simulink model "pattern3x3_training_2023clock"  (R2024a)
settings: Solver=FixedStepAuto  StartTime=0.0  StopTime=2  FixedStep=0.000005  RelTol=1e-3
model workspace (MAT data in the model file):
  part1_v1 = 1
values from neighbouring files (symbols this model uses):
  full_pattern = load('Pattern4_250.CSV')    [model_setup4.m]
  max_weight2 = 255    [model_setup4.m]
  min_weight2 = 150    [model_setup4.m]
  Th_minus_count2 = 10    [model_setup4.m]    (also in model_setup_test.m = 5)
  Th_plus_count2 = 20    [model_setup4.m]    (also in model_setup_test.m)
libraries: simulink x1
(part 7 of 9)

== system pattern3x3_training_2023clock/Synapse33/Clock3 ==
  clock : Inport
  "Reset " : Inport  Port=2
  Memory2 : Memory
  NOT1 : Logic  Operator=NOT  IconShape=distinctive  AllPortsSameDT=off  OutDataTypeStr=boolean
  Product1 : Product
  Triggered Subsystem1 : Subsystem  TreatAsAtomicUnit=on
  T : Outport  VectorParamsAs1DForOutWhenUnconnected=off
  wires:
  Memory2/1 -> Triggered Subsystem1/1(In1)
  Product1/1 -> T/1, Memory2/1
  "Reset "/1 -> NOT1/1
  Triggered Subsystem1/1(Out1) -> Product1/1
  NOT1/1 -> Product1/2
  clock/1 -> Triggered Subsystem1/Trigger

== system pattern3x3_training_2023clock/Synapse33/Subsystem ==
  delta_weight : Inport
  before_weight : Inport  Port=2
  Trigger : TriggerPort  VariantControl=(inherit)  PortDimensions=1
  Sum : Sum  Inputs=|++
  weight : Outport
  wires:
  delta_weight/1 -> Sum/1
  Sum/1 -> weight/1
  before_weight/1 -> Sum/2

== system pattern3x3_training_2023clock/Synapse34/Clock1 ==
  clock : Inport
  "Reset " : Inport  Port=2
  Memory2 : Memory
  NOT1 : Logic  Operator=NOT  IconShape=distinctive  AllPortsSameDT=off  OutDataTypeStr=boolean
  Product1 : Product
  Triggered Subsystem1 : Subsystem  TreatAsAtomicUnit=on
  T : Outport  VectorParamsAs1DForOutWhenUnconnected=off
  wires:
  Memory2/1 -> Triggered Subsystem1/1(In1)
  Product1/1 -> T/1, Memory2/1
  "Reset "/1 -> NOT1/1
  Triggered Subsystem1/1(Out1) -> Product1/1
  NOT1/1 -> Product1/2
  clock/1 -> Triggered Subsystem1/Trigger

== system pattern3x3_training_2023clock/Synapse34/Clock2 ==
  clock : Inport
  "Reset " : Inport  Port=2
  Memory2 : Memory
  NOT1 : Logic  Operator=NOT  IconShape=distinctive  AllPortsSameDT=off  OutDataTypeStr=boolean
  Product1 : Product
  Triggered Subsystem1 : Subsystem  TreatAsAtomicUnit=on
  T : Outport  VectorParamsAs1DForOutWhenUnconnected=off
  wires:
  Memory2/1 -> Triggered Subsystem1/1(In1)
  Product1/1 -> T/1, Memory2/1
  "Reset "/1 -> NOT1/1
  Triggered Subsystem1/1(Out1) -> Product1/1
  NOT1/1 -> Product1/2
  clock/1 -> Triggered Subsystem1/Trigger

== system pattern3x3_training_2023clock/Synapse34/Clock3 ==
  clock : Inport
  "Reset " : Inport  Port=2
  Memory2 : Memory
  NOT1 : Logic  Operator=NOT  IconShape=distinctive  AllPortsSameDT=off  OutDataTypeStr=boolean
  Product1 : Product
  Triggered Subsystem1 : Subsystem  TreatAsAtomicUnit=on
  T : Outport  VectorParamsAs1DForOutWhenUnconnected=off
  wires:
  Memory2/1 -> Triggered Subsystem1/1(In1)
  Product1/1 -> T/1, Memory2/1
  "Reset "/1 -> NOT1/1
  Triggered Subsystem1/1(Out1) -> Product1/1
  NOT1/1 -> Product1/2
  clock/1 -> Triggered Subsystem1/Trigger

== system pattern3x3_training_2023clock/Synapse34/Subsystem ==
  delta_weight : Inport
  before_weight : Inport  Port=2
  Trigger : TriggerPort  VariantControl=(inherit)  PortDimensions=1
  Sum : Sum  Inputs=|++
  weight : Outport
  wires:
  delta_weight/1 -> Sum/1
  Sum/1 -> weight/1
  before_weight/1 -> Sum/2

== system pattern3x3_training_2023clock/Synapse35/Clock1 ==
  clock : Inport
  "Reset " : Inport  Port=2
  Memory2 : Memory
  NOT1 : Logic  Operator=NOT  IconShape=distinctive  AllPortsSameDT=off  OutDataTypeStr=boolean
  Product1 : Product
  Triggered Subsystem1 : Subsystem  TreatAsAtomicUnit=on
  T : Outport  VectorParamsAs1DForOutWhenUnconnected=off
  wires:
  Memory2/1 -> Triggered Subsystem1/1(In1)
  Product1/1 -> T/1, Memory2/1
  "Reset "/1 -> NOT1/1
  Triggered Subsystem1/1(Out1) -> Product1/1
  NOT1/1 -> Product1/2
  clock/1 -> Triggered Subsystem1/Trigger

== system pattern3x3_training_2023clock/Synapse35/Clock2 ==
  clock : Inport
  "Reset " : Inport  Port=2
  Memory2 : Memory
  NOT1 : Logic  Operator=NOT  IconShape=distinctive  AllPortsSameDT=off  OutDataTypeStr=boolean
  Product1 : Product
  Triggered Subsystem1 : Subsystem  TreatAsAtomicUnit=on
  T : Outport  VectorParamsAs1DForOutWhenUnconnected=off
  wires:
  Memory2/1 -> Triggered Subsystem1/1(In1)
  Product1/1 -> T/1, Memory2/1
  "Reset "/1 -> NOT1/1
  Triggered Subsystem1/1(Out1) -> Product1/1
  NOT1/1 -> Product1/2
  clock/1 -> Triggered Subsystem1/Trigger

== system pattern3x3_training_2023clock/Synapse35/Clock3 ==
  clock : Inport
  "Reset " : Inport  Port=2
  Memory2 : Memory
  NOT1 : Logic  Operator=NOT  IconShape=distinctive  AllPortsSameDT=off  OutDataTypeStr=boolean
  Product1 : Product
  Triggered Subsystem1 : Subsystem  TreatAsAtomicUnit=on
  T : Outport  VectorParamsAs1DForOutWhenUnconnected=off
  wires:
  Memory2/1 -> Triggered Subsystem1/1(In1)
  Product1/1 -> T/1, Memory2/1
  "Reset "/1 -> NOT1/1
  Triggered Subsystem1/1(Out1) -> Product1/1
  NOT1/1 -> Product1/2
  clock/1 -> Triggered Subsystem1/Trigger

== system pattern3x3_training_2023clock/Synapse35/Subsystem ==
  delta_weight : Inport
  before_weight : Inport  Port=2
  Trigger : TriggerPort  VariantControl=(inherit)  PortDimensions=1
  Sum : Sum  Inputs=|++
  weight : Outport
  wires:
  delta_weight/1 -> Sum/1
  Sum/1 -> weight/1
  before_weight/1 -> Sum/2

== system pattern3x3_training_2023clock/Synapse36/Clock1 ==
  clock : Inport
  "Reset " : Inport  Port=2
  Memory2 : Memory
  NOT1 : Logic  Operator=NOT  IconShape=distinctive  AllPortsSameDT=off  OutDataTypeStr=boolean
  Product1 : Product
  Triggered Subsystem1 : Subsystem  TreatAsAtomicUnit=on
  T : Outport  VectorParamsAs1DForOutWhenUnconnected=off
  wires:
  Memory2/1 -> Triggered Subsystem1/1(In1)
  Product1/1 -> T/1, Memory2/1
  "Reset "/1 -> NOT1/1
  Triggered Subsystem1/1(Out1) -> Product1/1
  NOT1/1 -> Product1/2
  clock/1 -> Triggered Subsystem1/Trigger

== system pattern3x3_training_2023clock/Synapse36/Clock2 ==
  clock : Inport
  "Reset " : Inport  Port=2
  Memory2 : Memory
  NOT1 : Logic  Operator=NOT  IconShape=distinctive  AllPortsSameDT=off  OutDataTypeStr=boolean
  Product1 : Product
  Triggered Subsystem1 : Subsystem  TreatAsAtomicUnit=on
  T : Outport  VectorParamsAs1DForOutWhenUnconnected=off
  wires:
  Memory2/1 -> Triggered Subsystem1/1(In1)
  Product1/1 -> T/1, Memory2/1
  "Reset "/1 -> NOT1/1
  Triggered Subsystem1/1(Out1) -> Product1/1
  NOT1/1 -> Product1/2
  clock/1 -> Triggered Subsystem1/Trigger

== system pattern3x3_training_2023clock/Synapse36/Clock3 ==
  clock : Inport
  "Reset " : Inport  Port=2
  Memory2 : Memory
  NOT1 : Logic  Operator=NOT  IconShape=distinctive  AllPortsSameDT=off  OutDataTypeStr=boolean
  Product1 : Product
  Triggered Subsystem1 : Subsystem  TreatAsAtomicUnit=on
  T : Outport  VectorParamsAs1DForOutWhenUnconnected=off
  wires:
  Memory2/1 -> Triggered Subsystem1/1(In1)
  Product1/1 -> T/1, Memory2/1
  "Reset "/1 -> NOT1/1
  Triggered Subsystem1/1(Out1) -> Product1/1
  NOT1/1 -> Product1/2
  clock/1 -> Triggered Subsystem1/Trigger

== system pattern3x3_training_2023clock/Synapse36/Subsystem ==
  delta_weight : Inport
  before_weight : Inport  Port=2
  Trigger : TriggerPort  VariantControl=(inherit)  PortDimensions=1
  Sum : Sum  Inputs=|++
  weight : Outport
  wires:
  delta_weight/1 -> Sum/1
  Sum/1 -> weight/1
  before_weight/1 -> Sum/2

== system pattern3x3_training_2023clock/Synapse4/Clock1 ==
  clock : Inport
  "Reset " : Inport  Port=2
  Memory2 : Memory
  NOT1 : Logic  Operator=NOT  IconShape=distinctive  AllPortsSameDT=off  OutDataTypeStr=boolean
  Product1 : Product
  Triggered Subsystem1 : Subsystem  TreatAsAtomicUnit=on
  T : Outport  VectorParamsAs1DForOutWhenUnconnected=off
  wires:
  Memory2/1 -> Triggered Subsystem1/1(In1)
  Product1/1 -> T/1, Memory2/1
  "Reset "/1 -> NOT1/1
  Triggered Subsystem1/1(Out1) -> Product1/1
  NOT1/1 -> Product1/2
  clock/1 -> Triggered Subsystem1/Trigger

== system pattern3x3_training_2023clock/Synapse4/Clock2 ==
  clock : Inport
  "Reset " : Inport  Port=2
  Memory2 : Memory
  NOT1 : Logic  Operator=NOT  IconShape=distinctive  AllPortsSameDT=off  OutDataTypeStr=boolean
  Product1 : Product
  Triggered Subsystem1 : Subsystem  TreatAsAtomicUnit=on
  T : Outport  VectorParamsAs1DForOutWhenUnconnected=off
  wires:
  Memory2/1 -> Triggered Subsystem1/1(In1)
  Product1/1 -> T/1, Memory2/1
  "Reset "/1 -> NOT1/1
  Triggered Subsystem1/1(Out1) -> Product1/1
  NOT1/1 -> Product1/2
  clock/1 -> Triggered Subsystem1/Trigger

== system pattern3x3_training_2023clock/Synapse4/Clock3 ==
  clock : Inport
  "Reset " : Inport  Port=2
  Memory2 : Memory
  NOT1 : Logic  Operator=NOT  IconShape=distinctive  AllPortsSameDT=off  OutDataTypeStr=boolean
  Product1 : Product
  Triggered Subsystem1 : Subsystem  TreatAsAtomicUnit=on
  T : Outport  VectorParamsAs1DForOutWhenUnconnected=off
  wires:
  Memory2/1 -> Triggered Subsystem1/1(In1)
  Product1/1 -> T/1, Memory2/1
  "Reset "/1 -> NOT1/1
  Triggered Subsystem1/1(Out1) -> Product1/1
  NOT1/1 -> Product1/2
  clock/1 -> Triggered Subsystem1/Trigger

== system pattern3x3_training_2023clock/Synapse4/Subsystem ==
  delta_weight : Inport
  before_weight : Inport  Port=2
  Trigger : TriggerPort  VariantControl=(inherit)  PortDimensions=1
  Sum : Sum  Inputs=|++
  weight : Outport
  wires:
  delta_weight/1 -> Sum/1
  Sum/1 -> weight/1
  before_weight/1 -> Sum/2

== system pattern3x3_training_2023clock/Synapse5/Clock1 ==
  clock : Inport
  "Reset " : Inport  Port=2
  Memory2 : Memory
  NOT1 : Logic  Operator=NOT  IconShape=distinctive  AllPortsSameDT=off  OutDataTypeStr=boolean
  Product1 : Product
  Triggered Subsystem1 : Subsystem  TreatAsAtomicUnit=on
  T : Outport  VectorParamsAs1DForOutWhenUnconnected=off
  wires:
  Memory2/1 -> Triggered Subsystem1/1(In1)
  Product1/1 -> T/1, Memory2/1
  "Reset "/1 -> NOT1/1
  Triggered Subsystem1/1(Out1) -> Product1/1
  NOT1/1 -> Product1/2
  clock/1 -> Triggered Subsystem1/Trigger

== system pattern3x3_training_2023clock/Synapse5/Clock2 ==
  clock : Inport
  "Reset " : Inport  Port=2
  Memory2 : Memory
  NOT1 : Logic  Operator=NOT  IconShape=distinctive  AllPortsSameDT=off  OutDataTypeStr=boolean
  Product1 : Product
  Triggered Subsystem1 : Subsystem  TreatAsAtomicUnit=on
  T : Outport  VectorParamsAs1DForOutWhenUnconnected=off
  wires:
  Memory2/1 -> Triggered Subsystem1/1(In1)
  Product1/1 -> T/1, Memory2/1
  "Reset "/1 -> NOT1/1
  Triggered Subsystem1/1(Out1) -> Product1/1
  NOT1/1 -> Product1/2
  clock/1 -> Triggered Subsystem1/Trigger

== system pattern3x3_training_2023clock/Synapse5/Clock3 ==
  clock : Inport
  "Reset " : Inport  Port=2
  Memory2 : Memory
  NOT1 : Logic  Operator=NOT  IconShape=distinctive  AllPortsSameDT=off  OutDataTypeStr=boolean
  Product1 : Product
  Triggered Subsystem1 : Subsystem  TreatAsAtomicUnit=on
  T : Outport  VectorParamsAs1DForOutWhenUnconnected=off
  wires:
  Memory2/1 -> Triggered Subsystem1/1(In1)
  Product1/1 -> T/1, Memory2/1
  "Reset "/1 -> NOT1/1
  Triggered Subsystem1/1(Out1) -> Product1/1
  NOT1/1 -> Product1/2
  clock/1 -> Triggered Subsystem1/Trigger

== system pattern3x3_training_2023clock/Synapse5/Subsystem ==
  delta_weight : Inport
  before_weight : Inport  Port=2
  Trigger : TriggerPort  VariantControl=(inherit)  PortDimensions=1
  Sum : Sum  Inputs=|++
  weight : Outport
  wires:
  delta_weight/1 -> Sum/1
  Sum/1 -> weight/1
  before_weight/1 -> Sum/2

== system pattern3x3_training_2023clock/Synapse6/Clock1 ==
  clock : Inport
  "Reset " : Inport  Port=2
  Memory2 : Memory
  NOT1 : Logic  Operator=NOT  IconShape=distinctive  AllPortsSameDT=off  OutDataTypeStr=boolean
  Product1 : Product
  Triggered Subsystem1 : Subsystem  TreatAsAtomicUnit=on
  T : Outport  VectorParamsAs1DForOutWhenUnconnected=off
  wires:
  Memory2/1 -> Triggered Subsystem1/1(In1)
  Product1/1 -> T/1, Memory2/1
  "Reset "/1 -> NOT1/1
  Triggered Subsystem1/1(Out1) -> Product1/1
  NOT1/1 -> Product1/2
  clock/1 -> Triggered Subsystem1/Trigger

== system pattern3x3_training_2023clock/Synapse6/Clock2 ==
  clock : Inport
  "Reset " : Inport  Port=2
  Memory2 : Memory
  NOT1 : Logic  Operator=NOT  IconShape=distinctive  AllPortsSameDT=off  OutDataTypeStr=boolean
  Product1 : Product
  Triggered Subsystem1 : Subsystem  TreatAsAtomicUnit=on
  T : Outport  VectorParamsAs1DForOutWhenUnconnected=off
  wires:
  Memory2/1 -> Triggered Subsystem1/1(In1)
  Product1/1 -> T/1, Memory2/1
  "Reset "/1 -> NOT1/1
  Triggered Subsystem1/1(Out1) -> Product1/1
  NOT1/1 -> Product1/2
  clock/1 -> Triggered Subsystem1/Trigger

== system pattern3x3_training_2023clock/Synapse6/Clock3 ==
  clock : Inport
  "Reset " : Inport  Port=2
  Memory2 : Memory
  NOT1 : Logic  Operator=NOT  IconShape=distinctive  AllPortsSameDT=off  OutDataTypeStr=boolean
  Product1 : Product
  Triggered Subsystem1 : Subsystem  TreatAsAtomicUnit=on
  T : Outport  VectorParamsAs1DForOutWhenUnconnected=off
  wires:
  Memory2/1 -> Triggered Subsystem1/1(In1)
  Product1/1 -> T/1, Memory2/1
  "Reset "/1 -> NOT1/1
  Triggered Subsystem1/1(Out1) -> Product1/1
  NOT1/1 -> Product1/2
  clock/1 -> Triggered Subsystem1/Trigger

== system pattern3x3_training_2023clock/Synapse6/Subsystem ==
  delta_weight : Inport
  before_weight : Inport  Port=2
  Trigger : TriggerPort  VariantControl=(inherit)  PortDimensions=1
  Sum : Sum  Inputs=|++
  weight : Outport
  wires:
  delta_weight/1 -> Sum/1
  Sum/1 -> weight/1
  before_weight/1 -> Sum/2

== system pattern3x3_training_2023clock/Synapse7/Clock1 ==
  clock : Inport
  "Reset " : Inport  Port=2
  Memory2 : Memory
  NOT1 : Logic  Operator=NOT  IconShape=distinctive  AllPortsSameDT=off  OutDataTypeStr=boolean
  Product1 : Product
  Triggered Subsystem1 : Subsystem  TreatAsAtomicUnit=on
  T : Outport  VectorParamsAs1DForOutWhenUnconnected=off
  wires:
  Memory2/1 -> Triggered Subsystem1/1(In1)
  Product1/1 -> T/1, Memory2/1
  "Reset "/1 -> NOT1/1
  Triggered Subsystem1/1(Out1) -> Product1/1
  NOT1/1 -> Product1/2
  clock/1 -> Triggered Subsystem1/Trigger

== system pattern3x3_training_2023clock/Synapse7/Clock2 ==
  clock : Inport
  "Reset " : Inport  Port=2
  Memory2 : Memory
  NOT1 : Logic  Operator=NOT  IconShape=distinctive  AllPortsSameDT=off  OutDataTypeStr=boolean
  Product1 : Product
  Triggered Subsystem1 : Subsystem  TreatAsAtomicUnit=on
  T : Outport  VectorParamsAs1DForOutWhenUnconnected=off
  wires:
  Memory2/1 -> Triggered Subsystem1/1(In1)
  Product1/1 -> T/1, Memory2/1
  "Reset "/1 -> NOT1/1
  Triggered Subsystem1/1(Out1) -> Product1/1
  NOT1/1 -> Product1/2
  clock/1 -> Triggered Subsystem1/Trigger

== system pattern3x3_training_2023clock/Synapse7/Clock3 ==
  clock : Inport
  "Reset " : Inport  Port=2
  Memory2 : Memory
  NOT1 : Logic  Operator=NOT  IconShape=distinctive  AllPortsSameDT=off  OutDataTypeStr=boolean
  Product1 : Product
  Triggered Subsystem1 : Subsystem  TreatAsAtomicUnit=on
  T : Outport  VectorParamsAs1DForOutWhenUnconnected=off
  wires:
  Memory2/1 -> Triggered Subsystem1/1(In1)
  Product1/1 -> T/1, Memory2/1
  "Reset "/1 -> NOT1/1
  Triggered Subsystem1/1(Out1) -> Product1/1
  NOT1/1 -> Product1/2
  clock/1 -> Triggered Subsystem1/Trigger

== system pattern3x3_training_2023clock/Synapse7/Subsystem ==
  delta_weight : Inport
  before_weight : Inport  Port=2
  Trigger : TriggerPort  VariantControl=(inherit)  PortDimensions=1
  Sum : Sum  Inputs=|++
  weight : Outport
  wires:
  delta_weight/1 -> Sum/1
  Sum/1 -> weight/1
  before_weight/1 -> Sum/2

== system pattern3x3_training_2023clock/Synapse8/Clock1 ==
  clock : Inport
  "Reset " : Inport  Port=2
  Memory2 : Memory
  NOT1 : Logic  Operator=NOT  IconShape=distinctive  AllPortsSameDT=off  OutDataTypeStr=boolean
  Product1 : Product
  Triggered Subsystem1 : Subsystem  TreatAsAtomicUnit=on
  T : Outport  VectorParamsAs1DForOutWhenUnconnected=off
  wires:
  Memory2/1 -> Triggered Subsystem1/1(In1)
  Product1/1 -> T/1, Memory2/1
  "Reset "/1 -> NOT1/1
  Triggered Subsystem1/1(Out1) -> Product1/1
  NOT1/1 -> Product1/2
  clock/1 -> Triggered Subsystem1/Trigger

== system pattern3x3_training_2023clock/Synapse8/Clock2 ==
  clock : Inport
  "Reset " : Inport  Port=2
  Memory2 : Memory
  NOT1 : Logic  Operator=NOT  IconShape=distinctive  AllPortsSameDT=off  OutDataTypeStr=boolean
  Product1 : Product
  Triggered Subsystem1 : Subsystem  TreatAsAtomicUnit=on
  T : Outport  VectorParamsAs1DForOutWhenUnconnected=off
  wires:
  Memory2/1 -> Triggered Subsystem1/1(In1)
  Product1/1 -> T/1, Memory2/1
  "Reset "/1 -> NOT1/1
  Triggered Subsystem1/1(Out1) -> Product1/1
  NOT1/1 -> Product1/2
  clock/1 -> Triggered Subsystem1/Trigger

== system pattern3x3_training_2023clock/Synapse8/Clock3 ==
  clock : Inport
  "Reset " : Inport  Port=2
  Memory2 : Memory
  NOT1 : Logic  Operator=NOT  IconShape=distinctive  AllPortsSameDT=off  OutDataTypeStr=boolean
  Product1 : Product
  Triggered Subsystem1 : Subsystem  TreatAsAtomicUnit=on
  T : Outport  VectorParamsAs1DForOutWhenUnconnected=off
  wires:
  Memory2/1 -> Triggered Subsystem1/1(In1)
  Product1/1 -> T/1, Memory2/1
  "Reset "/1 -> NOT1/1
  Triggered Subsystem1/1(Out1) -> Product1/1
  NOT1/1 -> Product1/2
  clock/1 -> Triggered Subsystem1/Trigger

== system pattern3x3_training_2023clock/Synapse8/Subsystem ==
  delta_weight : Inport
  before_weight : Inport  Port=2
  Trigger : TriggerPort  VariantControl=(inherit)  PortDimensions=1
  Sum : Sum  Inputs=|++
  weight : Outport
  wires:
  delta_weight/1 -> Sum/1
  Sum/1 -> weight/1
  before_weight/1 -> Sum/2

== system pattern3x3_training_2023clock/Synapse9/Clock1 ==
  clock : Inport
  "Reset " : Inport  Port=2
  Memory2 : Memory
  NOT1 : Logic  Operator=NOT  IconShape=distinctive  AllPortsSameDT=off  OutDataTypeStr=boolean
  Product1 : Product
  Triggered Subsystem1 : Subsystem  TreatAsAtomicUnit=on
  T : Outport  VectorParamsAs1DForOutWhenUnconnected=off
  wires:
  Memory2/1 -> Triggered Subsystem1/1(In1)
  Product1/1 -> T/1, Memory2/1
  "Reset "/1 -> NOT1/1
  Triggered Subsystem1/1(Out1) -> Product1/1
  NOT1/1 -> Product1/2
  clock/1 -> Triggered Subsystem1/Trigger

== system pattern3x3_training_2023clock/Synapse9/Clock2 ==
  clock : Inport
  "Reset " : Inport  Port=2
  Memory2 : Memory
  NOT1 : Logic  Operator=NOT  IconShape=distinctive  AllPortsSameDT=off  OutDataTypeStr=boolean
  Product1 : Product
  Triggered Subsystem1 : Subsystem  TreatAsAtomicUnit=on
  T : Outport  VectorParamsAs1DForOutWhenUnconnected=off
  wires:
  Memory2/1 -> Triggered Subsystem1/1(In1)
  Product1/1 -> T/1, Memory2/1
  "Reset "/1 -> NOT1/1
  Triggered Subsystem1/1(Out1) -> Product1/1
  NOT1/1 -> Product1/2
  clock/1 -> Triggered Subsystem1/Trigger

== system pattern3x3_training_2023clock/Synapse9/Clock3 ==
  clock : Inport
  "Reset " : Inport  Port=2
  Memory2 : Memory
  NOT1 : Logic  Operator=NOT  IconShape=distinctive  AllPortsSameDT=off  OutDataTypeStr=boolean
  Product1 : Product
  Triggered Subsystem1 : Subsystem  TreatAsAtomicUnit=on
  T : Outport  VectorParamsAs1DForOutWhenUnconnected=off
  wires:
  Memory2/1 -> Triggered Subsystem1/1(In1)
  Product1/1 -> T/1, Memory2/1
  "Reset "/1 -> NOT1/1
  Triggered Subsystem1/1(Out1) -> Product1/1
  NOT1/1 -> Product1/2
  clock/1 -> Triggered Subsystem1/Trigger

== system pattern3x3_training_2023clock/Synapse9/Subsystem ==
  delta_weight : Inport
  before_weight : Inport  Port=2
  Trigger : TriggerPort  VariantControl=(inherit)  PortDimensions=1
  Sum : Sum  Inputs=|++
  weight : Outport
  wires:
  delta_weight/1 -> Sum/1
  Sum/1 -> weight/1
  before_weight/1 -> Sum/2

== system pattern3x3_training_2023clock/clock_0.001/Triggered Subsystem1 ==
  In1 : Inport
  Trigger : TriggerPort  VariantControl=Variant
  Constant : Constant
  Sum : Sum  Inputs=|++
  Out1 : Outport  VectorParamsAs1DForOutWhenUnconnected=off
  wires:
  Constant/1 -> Sum/2
  In1/1 -> Sum/1
  Sum/1 -> Out1/1

== system pattern3x3_training_2023clock/Neuron1/Clock4/Triggered Subsystem1 ==
  In1 : Inport
  Trigger : TriggerPort  VariantControl=Variant
  Constant : Constant
  Sum : Sum  Inputs=|++
  Out1 : Outport  VectorParamsAs1DForOutWhenUnconnected=off
  wires:
  Constant/1 -> Sum/2
  In1/1 -> Sum/1
  Sum/1 -> Out1/1

== system pattern3x3_training_2023clock/Neuron1/Subsystem3/clock_0.02 ==
  In1 : Inport
  Memory1 : Memory
  Memory3 : Memory
  Multiply : Gain  Gain=0.0005
  NOT1 : Logic  Operator=NOT  IconShape=distinctive  AllPortsSameDT=off  OutDataTypeStr=boolean
  OR : Logic  Operator=OR  IconShape=distinctive  AllPortsSameDT=off  OutDataTypeStr=boolean
  One : Constant  OutDataTypeStr=Inherit: Inherit via back propagation
  Product1 : Product
  Scope4 : Scope  NumInputPorts=4
  Switch1 : Switch  Threshold=1  SaturateOnIntegerOverflow=off  InputSameDT=off
  Triggered Subsystem1 : Subsystem  TreatAsAtomicUnit=on
  Zero : Constant  Value=0  OutDataTypeStr=Inherit: Inherit via back propagation
  clock : Outport
  wires:
  Product1/1 -> Multiply/1, Memory1/1, Scope4/2
  One/1 -> Switch1/1
  Multiply/1 -> Switch1/2
  Triggered Subsystem1/1(Out1) -> Product1/1
  In1/1 -> Triggered Subsystem1/Trigger, Scope4/1
  Zero/1 -> Switch1/3
  NOT1/1 -> Product1/2
  Memory3/1 -> OR/2, NOT1/1
  Memory1/1 -> Triggered Subsystem1/1(In1)
  OR/1 -> Scope4/4, clock/1
  Switch1/1 -> Scope4/3, Memory3/1, OR/1

== system pattern3x3_training_2023clock/Neuron1/Subsystem3/spike_generator2 ==
  del_th : Inport
  AND : Logic  IconShape=distinctive  AllPortsSameDT=off  OutDataTypeStr=boolean
  Delay1 : Delay  DelayLength=1  SampleTime=0.00001
  NOT : Logic  Operator=NOT  IconShape=distinctive  AllPortsSameDT=off  OutDataTypeStr=boolean
  Product : Product
  del_th_spike : Outport
  wires:
  NOT/1 -> Delay1/1
  AND/1 -> Product/1
  Delay1/1 -> AND/2
  Product/1 -> del_th_spike/1
  del_th/1 -> AND/1, Product/2, NOT/1

== system pattern3x3_training_2023clock/Neuron2/Clock4/Triggered Subsystem1 ==
  In1 : Inport
  Trigger : TriggerPort  VariantControl=Variant
  Constant : Constant
  Sum : Sum  Inputs=|++
  Out1 : Outport  VectorParamsAs1DForOutWhenUnconnected=off
  wires:
  Constant/1 -> Sum/2
  In1/1 -> Sum/1
  Sum/1 -> Out1/1

== system pattern3x3_training_2023clock/Neuron2/Subsystem3/clock_0.02 ==
  In1 : Inport
  Memory1 : Memory
  Memory3 : Memory
  Multiply : Gain  Gain=0.0005
  NOT1 : Logic  Operator=NOT  IconShape=distinctive  AllPortsSameDT=off  OutDataTypeStr=boolean
  OR : Logic  Operator=OR  IconShape=distinctive  AllPortsSameDT=off  OutDataTypeStr=boolean
  One : Constant  OutDataTypeStr=Inherit: Inherit via back propagation
  Product1 : Product
  Scope4 : Scope  NumInputPorts=4
  Switch1 : Switch  Threshold=1  SaturateOnIntegerOverflow=off  InputSameDT=off
  Triggered Subsystem1 : Subsystem  TreatAsAtomicUnit=on
  Zero : Constant  Value=0  OutDataTypeStr=Inherit: Inherit via back propagation
  clock : Outport
  wires:
  Product1/1 -> Multiply/1, Memory1/1, Scope4/2
  One/1 -> Switch1/1
  Multiply/1 -> Switch1/2
  Triggered Subsystem1/1(Out1) -> Product1/1
  In1/1 -> Triggered Subsystem1/Trigger, Scope4/1
  Zero/1 -> Switch1/3
  NOT1/1 -> Product1/2
  Memory3/1 -> OR/2, NOT1/1
  Memory1/1 -> Triggered Subsystem1/1(In1)
  OR/1 -> Scope4/4, clock/1
  Switch1/1 -> Scope4/3, Memory3/1, OR/1

== system pattern3x3_training_2023clock/Neuron2/Subsystem3/spike_generator2 ==
  del_th : Inport
  AND : Logic  IconShape=distinctive  AllPortsSameDT=off  OutDataTypeStr=boolean
  Delay1 : Delay  DelayLength=1  SampleTime=0.00001
  NOT : Logic  Operator=NOT  IconShape=distinctive  AllPortsSameDT=off  OutDataTypeStr=boolean
  Product : Product
  del_th_spike : Outport
  wires:
  NOT/1 -> Delay1/1
  AND/1 -> Product/1
  Delay1/1 -> AND/2
  Product/1 -> del_th_spike/1
  del_th/1 -> AND/1, Product/2, NOT/1

== system pattern3x3_training_2023clock/Neuron3/Clock4/Triggered Subsystem1 ==
  In1 : Inport
  Trigger : TriggerPort  VariantControl=Variant
  Constant : Constant
  Sum : Sum  Inputs=|++
  Out1 : Outport  VectorParamsAs1DForOutWhenUnconnected=off
  wires:
  Constant/1 -> Sum/2
  In1/1 -> Sum/1
  Sum/1 -> Out1/1

== system pattern3x3_training_2023clock/Neuron3/Subsystem3/clock_0.02 ==
  In1 : Inport
  Memory1 : Memory
  Memory3 : Memory
  Multiply : Gain  Gain=0.0005
  NOT1 : Logic  Operator=NOT  IconShape=distinctive  AllPortsSameDT=off  OutDataTypeStr=boolean
  OR : Logic  Operator=OR  IconShape=distinctive  AllPortsSameDT=off  OutDataTypeStr=boolean
  One : Constant  OutDataTypeStr=Inherit: Inherit via back propagation
  Product1 : Product
  Scope4 : Scope  NumInputPorts=4
  Switch1 : Switch  Threshold=1  SaturateOnIntegerOverflow=off  InputSameDT=off
  Triggered Subsystem1 : Subsystem  TreatAsAtomicUnit=on
  Zero : Constant  Value=0  OutDataTypeStr=Inherit: Inherit via back propagation
  clock : Outport
  wires:
  Product1/1 -> Multiply/1, Memory1/1, Scope4/2
  One/1 -> Switch1/1
  Multiply/1 -> Switch1/2
  Triggered Subsystem1/1(Out1) -> Product1/1
  In1/1 -> Triggered Subsystem1/Trigger, Scope4/1
  Zero/1 -> Switch1/3
  NOT1/1 -> Product1/2
  Memory3/1 -> OR/2, NOT1/1
  Memory1/1 -> Triggered Subsystem1/1(In1)
  OR/1 -> Scope4/4, clock/1
  Switch1/1 -> Scope4/3, Memory3/1, OR/1

== system pattern3x3_training_2023clock/Neuron3/Subsystem3/spike_generator2 ==
  del_th : Inport
  AND : Logic  IconShape=distinctive  AllPortsSameDT=off  OutDataTypeStr=boolean
  Delay1 : Delay  DelayLength=1  SampleTime=0.00001
  NOT : Logic  Operator=NOT  IconShape=distinctive  AllPortsSameDT=off  OutDataTypeStr=boolean
  Product : Product
  del_th_spike : Outport
  wires:
  NOT/1 -> Delay1/1
  AND/1 -> Product/1
  Delay1/1 -> AND/2
  Product/1 -> del_th_spike/1
  del_th/1 -> AND/1, Product/2, NOT/1

== system pattern3x3_training_2023clock/Neuron4/Clock4/Triggered Subsystem1 ==
  In1 : Inport
  Trigger : TriggerPort  VariantControl=Variant
  Constant : Constant
  Sum : Sum  Inputs=|++
  Out1 : Outport  VectorParamsAs1DForOutWhenUnconnected=off
  wires:
  Constant/1 -> Sum/2
  In1/1 -> Sum/1
  Sum/1 -> Out1/1

== system pattern3x3_training_2023clock/Neuron4/Subsystem3/clock_0.02 ==
  In1 : Inport
  Memory1 : Memory
  Memory3 : Memory
  Multiply : Gain  Gain=0.0005
  NOT1 : Logic  Operator=NOT  IconShape=distinctive  AllPortsSameDT=off  OutDataTypeStr=boolean
  OR : Logic  Operator=OR  IconShape=distinctive  AllPortsSameDT=off  OutDataTypeStr=boolean
  One : Constant  OutDataTypeStr=Inherit: Inherit via back propagation
  Product1 : Product
  Scope4 : Scope  NumInputPorts=4
  Switch1 : Switch  Threshold=1  SaturateOnIntegerOverflow=off  InputSameDT=off
  Triggered Subsystem1 : Subsystem  TreatAsAtomicUnit=on
  Zero : Constant  Value=0  OutDataTypeStr=Inherit: Inherit via back propagation
  clock : Outport
  wires:
  Product1/1 -> Multiply/1, Memory1/1, Scope4/2
  One/1 -> Switch1/1
  Multiply/1 -> Switch1/2
  Triggered Subsystem1/1(Out1) -> Product1/1
  In1/1 -> Triggered Subsystem1/Trigger, Scope4/1
  Zero/1 -> Switch1/3
  NOT1/1 -> Product1/2
  Memory3/1 -> OR/2, NOT1/1
  Memory1/1 -> Triggered Subsystem1/1(In1)
  OR/1 -> Scope4/4, clock/1
  Switch1/1 -> Scope4/3, Memory3/1, OR/1

== system pattern3x3_training_2023clock/Neuron4/Subsystem3/spike_generator2 ==
  del_th : Inport
  AND : Logic  IconShape=distinctive  AllPortsSameDT=off  OutDataTypeStr=boolean
  Delay1 : Delay  DelayLength=1  SampleTime=0.00001
  NOT : Logic  Operator=NOT  IconShape=distinctive  AllPortsSameDT=off  OutDataTypeStr=boolean
  Product : Product
  del_th_spike : Outport
  wires:
  NOT/1 -> Delay1/1
  AND/1 -> Product/1
  Delay1/1 -> AND/2
  Product/1 -> del_th_spike/1
  del_th/1 -> AND/1, Product/2, NOT/1

== system pattern3x3_training_2023clock/Neuron5/Clock4/Triggered Subsystem1 ==
  In1 : Inport
  Trigger : TriggerPort  VariantControl=Variant
  Constant : Constant
  Sum : Sum  Inputs=|++
  Out1 : Outport  VectorParamsAs1DForOutWhenUnconnected=off
  wires:
  Constant/1 -> Sum/2
  In1/1 -> Sum/1
  Sum/1 -> Out1/1

== system pattern3x3_training_2023clock/Neuron5/Subsystem3/clock_0.02 ==
  In1 : Inport
  Memory1 : Memory
  Memory3 : Memory
  Multiply : Gain  Gain=0.0005
  NOT1 : Logic  Operator=NOT  IconShape=distinctive  AllPortsSameDT=off  OutDataTypeStr=boolean
  OR : Logic  Operator=OR  IconShape=distinctive  AllPortsSameDT=off  OutDataTypeStr=boolean
  One : Constant  OutDataTypeStr=Inherit: Inherit via back propagation
  Product1 : Product
  Scope4 : Scope  NumInputPorts=4
  Switch1 : Switch  Threshold=1  SaturateOnIntegerOverflow=off  InputSameDT=off
  Triggered Subsystem1 : Subsystem  TreatAsAtomicUnit=on
  Zero : Constant  Value=0  OutDataTypeStr=Inherit: Inherit via back propagation
  clock : Outport
  wires:
  Product1/1 -> Multiply/1, Memory1/1, Scope4/2
  One/1 -> Switch1/1
  Multiply/1 -> Switch1/2
  Triggered Subsystem1/1(Out1) -> Product1/1
  In1/1 -> Triggered Subsystem1/Trigger, Scope4/1
  Zero/1 -> Switch1/3
  NOT1/1 -> Product1/2
  Memory3/1 -> OR/2, NOT1/1
  Memory1/1 -> Triggered Subsystem1/1(In1)
  OR/1 -> Scope4/4, clock/1
  Switch1/1 -> Scope4/3, Memory3/1, OR/1

== system pattern3x3_training_2023clock/Neuron5/Subsystem3/spike_generator2 ==
  del_th : Inport
  AND : Logic  IconShape=distinctive  AllPortsSameDT=off  OutDataTypeStr=boolean
  Delay1 : Delay  DelayLength=1  SampleTime=0.00001
  NOT : Logic  Operator=NOT  IconShape=distinctive  AllPortsSameDT=off  OutDataTypeStr=boolean
  Product : Product
  del_th_spike : Outport
  wires:
  NOT/1 -> Delay1/1
  AND/1 -> Product/1
  Delay1/1 -> AND/2
  Product/1 -> del_th_spike/1
  del_th/1 -> AND/1, Product/2, NOT/1

== system pattern3x3_training_2023clock/Neuron6/Clock4/Triggered Subsystem1 ==
  In1 : Inport
  Trigger : TriggerPort  VariantControl=Variant
  Constant : Constant
  Sum : Sum  Inputs=|++
  Out1 : Outport  VectorParamsAs1DForOutWhenUnconnected=off
  wires:
  Constant/1 -> Sum/2
  In1/1 -> Sum/1
  Sum/1 -> Out1/1

== system pattern3x3_training_2023clock/Neuron6/Subsystem3/clock_0.02 ==
  In1 : Inport
  Memory1 : Memory
  Memory3 : Memory
  Multiply : Gain  Gain=0.0005
  NOT1 : Logic  Operator=NOT  IconShape=distinctive  AllPortsSameDT=off  OutDataTypeStr=boolean
  OR : Logic  Operator=OR  IconShape=distinctive  AllPortsSameDT=off  OutDataTypeStr=boolean
  One : Constant  OutDataTypeStr=Inherit: Inherit via back propagation
  Product1 : Product
  Scope4 : Scope  NumInputPorts=4
  Switch1 : Switch  Threshold=1  SaturateOnIntegerOverflow=off  InputSameDT=off
  Triggered Subsystem1 : Subsystem  TreatAsAtomicUnit=on
  Zero : Constant  Value=0  OutDataTypeStr=Inherit: Inherit via back propagation
  clock : Outport
  wires:
  Product1/1 -> Multiply/1, Memory1/1, Scope4/2
  One/1 -> Switch1/1
  Multiply/1 -> Switch1/2
  Triggered Subsystem1/1(Out1) -> Product1/1
  In1/1 -> Triggered Subsystem1/Trigger, Scope4/1
  Zero/1 -> Switch1/3
  NOT1/1 -> Product1/2
  Memory3/1 -> OR/2, NOT1/1
  Memory1/1 -> Triggered Subsystem1/1(In1)
  OR/1 -> Scope4/4, clock/1
  Switch1/1 -> Scope4/3, Memory3/1, OR/1

== system pattern3x3_training_2023clock/Neuron6/Subsystem3/spike_generator2 ==
  del_th : Inport
  AND : Logic  IconShape=distinctive  AllPortsSameDT=off  OutDataTypeStr=boolean
  Delay1 : Delay  DelayLength=1  SampleTime=0.00001
  NOT : Logic  Operator=NOT  IconShape=distinctive  AllPortsSameDT=off  OutDataTypeStr=boolean
  Product : Product
  del_th_spike : Outport
  wires:
  NOT/1 -> Delay1/1
  AND/1 -> Product/1
  Delay1/1 -> AND/2
  Product/1 -> del_th_spike/1
  del_th/1 -> AND/1, Product/2, NOT/1

== system pattern3x3_training_2023clock/Neuron7/Clock4/Triggered Subsystem1 ==
  In1 : Inport
  Trigger : TriggerPort  VariantControl=Variant
  Constant : Constant
  Sum : Sum  Inputs=|++
  Out1 : Outport  VectorParamsAs1DForOutWhenUnconnected=off
  wires:
  Constant/1 -> Sum/2
  In1/1 -> Sum/1
  Sum/1 -> Out1/1

== system pattern3x3_training_2023clock/Neuron7/Subsystem3/clock_0.02 ==
  In1 : Inport
  Memory1 : Memory
  Memory3 : Memory
  Multiply : Gain  Gain=0.0005
  NOT1 : Logic  Operator=NOT  IconShape=distinctive  AllPortsSameDT=off  OutDataTypeStr=boolean
  OR : Logic  Operator=OR  IconShape=distinctive  AllPortsSameDT=off  OutDataTypeStr=boolean
  One : Constant  OutDataTypeStr=Inherit: Inherit via back propagation
  Product1 : Product
  Scope4 : Scope  NumInputPorts=4
  Switch1 : Switch  Threshold=1  SaturateOnIntegerOverflow=off  InputSameDT=off
  Triggered Subsystem1 : Subsystem  TreatAsAtomicUnit=on
  Zero : Constant  Value=0  OutDataTypeStr=Inherit: Inherit via back propagation
  clock : Outport
  wires:
  Product1/1 -> Multiply/1, Memory1/1, Scope4/2
  One/1 -> Switch1/1
  Multiply/1 -> Switch1/2
  Triggered Subsystem1/1(Out1) -> Product1/1
  In1/1 -> Triggered Subsystem1/Trigger, Scope4/1
  Zero/1 -> Switch1/3
  NOT1/1 -> Product1/2
  Memory3/1 -> OR/2, NOT1/1
  Memory1/1 -> Triggered Subsystem1/1(In1)
  OR/1 -> Scope4/4, clock/1
  Switch1/1 -> Scope4/3, Memory3/1, OR/1

== system pattern3x3_training_2023clock/Neuron7/Subsystem3/spike_generator2 ==
  del_th : Inport
  AND : Logic  IconShape=distinctive  AllPortsSameDT=off  OutDataTypeStr=boolean
  Delay1 : Delay  DelayLength=1  SampleTime=0.00001
  NOT : Logic  Operator=NOT  IconShape=distinctive  AllPortsSameDT=off  OutDataTypeStr=boolean
  Product : Product
  del_th_spike : Outport
  wires:
  NOT/1 -> Delay1/1
  AND/1 -> Product/1
  Delay1/1 -> AND/2
  Product/1 -> del_th_spike/1
  del_th/1 -> AND/1, Product/2, NOT/1

== system pattern3x3_training_2023clock/Neuron8/Clock4/Triggered Subsystem1 ==
  In1 : Inport
  Trigger : TriggerPort  VariantControl=Variant
  Constant : Constant
  Sum : Sum  Inputs=|++
  Out1 : Outport  VectorParamsAs1DForOutWhenUnconnected=off
  wires:
  Constant/1 -> Sum/2
  In1/1 -> Sum/1
  Sum/1 -> Out1/1

== system pattern3x3_training_2023clock/Neuron8/Subsystem3/clock_0.02 ==
  In1 : Inport
  Memory1 : Memory
  Memory3 : Memory
  Multiply : Gain  Gain=0.0005
  NOT1 : Logic  Operator=NOT  IconShape=distinctive  AllPortsSameDT=off  OutDataTypeStr=boolean
  OR : Logic  Operator=OR  IconShape=distinctive  AllPortsSameDT=off  OutDataTypeStr=boolean
  One : Constant  OutDataTypeStr=Inherit: Inherit via back propagation
  Product1 : Product
  Scope4 : Scope  NumInputPorts=4
  Switch1 : Switch  Threshold=1  SaturateOnIntegerOverflow=off  InputSameDT=off
  Triggered Subsystem1 : Subsystem  TreatAsAtomicUnit=on
  Zero : Constant  Value=0  OutDataTypeStr=Inherit: Inherit via back propagation
  clock : Outport
  wires:
  Product1/1 -> Multiply/1, Memory1/1, Scope4/2
  One/1 -> Switch1/1
  Multiply/1 -> Switch1/2
  Triggered Subsystem1/1(Out1) -> Product1/1
  In1/1 -> Triggered Subsystem1/Trigger, Scope4/1
  Zero/1 -> Switch1/3
  NOT1/1 -> Product1/2
  Memory3/1 -> OR/2, NOT1/1
  Memory1/1 -> Triggered Subsystem1/1(In1)
  OR/1 -> Scope4/4, clock/1
  Switch1/1 -> Scope4/3, Memory3/1, OR/1

== system pattern3x3_training_2023clock/Neuron8/Subsystem3/spike_generator2 ==
  del_th : Inport
  AND : Logic  IconShape=distinctive  AllPortsSameDT=off  OutDataTypeStr=boolean
  Delay1 : Delay  DelayLength=1  SampleTime=0.00001
  NOT : Logic  Operator=NOT  IconShape=distinctive  AllPortsSameDT=off  OutDataTypeStr=boolean
  Product : Product
  del_th_spike : Outport
  wires:
  NOT/1 -> Delay1/1
  AND/1 -> Product/1
  Delay1/1 -> AND/2
  Product/1 -> del_th_spike/1
  del_th/1 -> AND/1, Product/2, NOT/1

== system pattern3x3_training_2023clock/Neuron9/Clock4/Triggered Subsystem1 ==
  In1 : Inport
  Trigger : TriggerPort  VariantControl=Variant
  Constant : Constant
  Sum : Sum  Inputs=|++
  Out1 : Outport  VectorParamsAs1DForOutWhenUnconnected=off
  wires:
  Constant/1 -> Sum/2
  In1/1 -> Sum/1
  Sum/1 -> Out1/1

== system pattern3x3_training_2023clock/Neuron9/Subsystem3/clock_0.02 ==
  In1 : Inport
  Memory1 : Memory
  Memory3 : Memory
  Multiply : Gain  Gain=0.0005
  NOT1 : Logic  Operator=NOT  IconShape=distinctive  AllPortsSameDT=off  OutDataTypeStr=boolean
  OR : Logic  Operator=OR  IconShape=distinctive  AllPortsSameDT=off  OutDataTypeStr=boolean
  One : Constant  OutDataTypeStr=Inherit: Inherit via back propagation
  Product1 : Product
  Scope4 : Scope  NumInputPorts=4
  Switch1 : Switch  Threshold=1  SaturateOnIntegerOverflow=off  InputSameDT=off
  Triggered Subsystem1 : Subsystem  TreatAsAtomicUnit=on
  Zero : Constant  Value=0  OutDataTypeStr=Inherit: Inherit via back propagation
  clock : Outport
  wires:
  Product1/1 -> Multiply/1, Memory1/1, Scope4/2
  One/1 -> Switch1/1
  Multiply/1 -> Switch1/2
  Triggered Subsystem1/1(Out1) -> Product1/1
  In1/1 -> Triggered Subsystem1/Trigger, Scope4/1
  Zero/1 -> Switch1/3
  NOT1/1 -> Product1/2
  Memory3/1 -> OR/2, NOT1/1
  Memory1/1 -> Triggered Subsystem1/1(In1)
  OR/1 -> Scope4/4, clock/1
  Switch1/1 -> Scope4/3, Memory3/1, OR/1

== system pattern3x3_training_2023clock/Neuron9/Subsystem3/spike_generator2 ==
  del_th : Inport
  AND : Logic  IconShape=distinctive  AllPortsSameDT=off  OutDataTypeStr=boolean
  Delay1 : Delay  DelayLength=1  SampleTime=0.00001
  NOT : Logic  Operator=NOT  IconShape=distinctive  AllPortsSameDT=off  OutDataTypeStr=boolean
  Product : Product
  del_th_spike : Outport
  wires:
  NOT/1 -> Delay1/1
  AND/1 -> Product/1
  Delay1/1 -> AND/2
  Product/1 -> del_th_spike/1
  del_th/1 -> AND/1, Product/2, NOT/1

== system pattern3x3_training_2023clock/Post_Neuron1/Clock1/Triggered Subsystem1 ==
  In1 : Inport
  Trigger : TriggerPort  VariantControl=Variant
  Constant : Constant
  Sum : Sum  Inputs=|++
  Out1 : Outport  VectorParamsAs1DForOutWhenUnconnected=off
  wires:
  Constant/1 -> Sum/2
  In1/1 -> Sum/1
  Sum/1 -> Out1/1

== system pattern3x3_training_2023clock/Post_Neuron1/Clock2/Triggered Subsystem1 ==
  In1 : Inport
  Trigger : TriggerPort  VariantControl=Variant
  Constant : Constant
  Sum : Sum  Inputs=|++
  Out1 : Outport  VectorParamsAs1DForOutWhenUnconnected=off
  wires:
  Constant/1 -> Sum/2
  In1/1 -> Sum/1
  Sum/1 -> Out1/1

== system pattern3x3_training_2023clock/Post_Neuron1/Subsystem3/clock_0.02 ==
  In1 : Inport
  Memory1 : Memory
  Memory3 : Memory
  Multiply : Gain  Gain=0.0005
  NOT1 : Logic  Operator=NOT  IconShape=distinctive  AllPortsSameDT=off  OutDataTypeStr=boolean
  OR : Logic  Operator=OR  IconShape=distinctive  AllPortsSameDT=off  OutDataTypeStr=boolean
  One : Constant  OutDataTypeStr=Inherit: Inherit via back propagation
  Product1 : Product
  Scope4 : Scope  NumInputPorts=4
  Switch1 : Switch  Threshold=1  SaturateOnIntegerOverflow=off  InputSameDT=off
  Triggered Subsystem1 : Subsystem  TreatAsAtomicUnit=on
  Zero : Constant  Value=0  OutDataTypeStr=Inherit: Inherit via back propagation
  clock : Outport
  wires:
  Product1/1 -> Multiply/1, Memory1/1, Scope4/2
  One/1 -> Switch1/1
  Multiply/1 -> Switch1/2
  Triggered Subsystem1/1(Out1) -> Product1/1
  In1/1 -> Triggered Subsystem1/Trigger, Scope4/1
  Zero/1 -> Switch1/3
  NOT1/1 -> Product1/2
  Memory3/1 -> OR/2, NOT1/1
  Memory1/1 -> Triggered Subsystem1/1(In1)
  OR/1 -> Scope4/4, clock/1
  Switch1/1 -> Scope4/3, Memory3/1, OR/1

== system pattern3x3_training_2023clock/Post_Neuron1/Subsystem3/spike_generator2 ==
  del_th : Inport
  AND : Logic  IconShape=distinctive  AllPortsSameDT=off  OutDataTypeStr=boolean
  Delay1 : Delay  DelayLength=1  SampleTime=0.00001
  NOT : Logic  Operator=NOT  IconShape=distinctive  AllPortsSameDT=off  OutDataTypeStr=boolean
  Product : Product
  del_th_spike : Outport
  wires:
  NOT/1 -> Delay1/1
  AND/1 -> Product/1
  Delay1/1 -> AND/2
  Product/1 -> del_th_spike/1
  del_th/1 -> AND/1, Product/2, NOT/1

== system pattern3x3_training_2023clock/Post_Neuron2/Clock1/Triggered Subsystem1 ==
  In1 : Inport
  Trigger : TriggerPort  VariantControl=Variant
  Constant : Constant
  Sum : Sum  Inputs=|++
  Out1 : Outport  VectorParamsAs1DForOutWhenUnconnected=off
  wires:
  Constant/1 -> Sum/2
  In1/1 -> Sum/1
  Sum/1 -> Out1/1

== system pattern3x3_training_2023clock/Post_Neuron2/Clock2/Triggered Subsystem1 ==
  In1 : Inport
  Trigger : TriggerPort  VariantControl=Variant
  Constant : Constant
  Sum : Sum  Inputs=|++
  Out1 : Outport  VectorParamsAs1DForOutWhenUnconnected=off
  wires:
  Constant/1 -> Sum/2
  In1/1 -> Sum/1
  Sum/1 -> Out1/1

== system pattern3x3_training_2023clock/Post_Neuron2/Subsystem3/clock_0.02 ==
  In1 : Inport
  Memory1 : Memory
  Memory3 : Memory
  Multiply : Gain  Gain=0.0005
  NOT1 : Logic  Operator=NOT  IconShape=distinctive  AllPortsSameDT=off  OutDataTypeStr=boolean
  OR : Logic  Operator=OR  IconShape=distinctive  AllPortsSameDT=off  OutDataTypeStr=boolean
  One : Constant  OutDataTypeStr=Inherit: Inherit via back propagation
  Product1 : Product
  Scope4 : Scope  NumInputPorts=4
  Switch1 : Switch  Threshold=1  SaturateOnIntegerOverflow=off  InputSameDT=off
  Triggered Subsystem1 : Subsystem  TreatAsAtomicUnit=on
  Zero : Constant  Value=0  OutDataTypeStr=Inherit: Inherit via back propagation
  clock : Outport
  wires:
  Product1/1 -> Multiply/1, Memory1/1, Scope4/2
  One/1 -> Switch1/1
  Multiply/1 -> Switch1/2
  Triggered Subsystem1/1(Out1) -> Product1/1
  In1/1 -> Triggered Subsystem1/Trigger, Scope4/1
  Zero/1 -> Switch1/3
  NOT1/1 -> Product1/2
  Memory3/1 -> OR/2, NOT1/1
  Memory1/1 -> Triggered Subsystem1/1(In1)
  OR/1 -> Scope4/4, clock/1
  Switch1/1 -> Scope4/3, Memory3/1, OR/1

== system pattern3x3_training_2023clock/Post_Neuron2/Subsystem3/spike_generator2 ==
  del_th : Inport
  AND : Logic  IconShape=distinctive  AllPortsSameDT=off  OutDataTypeStr=boolean
  Delay1 : Delay  DelayLength=1  SampleTime=0.00001
  NOT : Logic  Operator=NOT  IconShape=distinctive  AllPortsSameDT=off  OutDataTypeStr=boolean
  Product : Product
  del_th_spike : Outport
  wires:
  NOT/1 -> Delay1/1
  AND/1 -> Product/1
  Delay1/1 -> AND/2
  Product/1 -> del_th_spike/1
  del_th/1 -> AND/1, Product/2, NOT/1

== system pattern3x3_training_2023clock/Post_Neuron3/Clock1/Triggered Subsystem1 ==
  In1 : Inport
  Trigger : TriggerPort  VariantControl=Variant
  Constant : Constant
  Sum : Sum  Inputs=|++
  Out1 : Outport  VectorParamsAs1DForOutWhenUnconnected=off
  wires:
  Constant/1 -> Sum/2
  In1/1 -> Sum/1
  Sum/1 -> Out1/1

== system pattern3x3_training_2023clock/Post_Neuron3/Clock2/Triggered Subsystem1 ==
  In1 : Inport
  Trigger : TriggerPort  VariantControl=Variant
  Constant : Constant
  Sum : Sum  Inputs=|++
  Out1 : Outport  VectorParamsAs1DForOutWhenUnconnected=off
  wires:
  Constant/1 -> Sum/2
  In1/1 -> Sum/1
  Sum/1 -> Out1/1

== system pattern3x3_training_2023clock/Post_Neuron3/Subsystem3/clock_0.02 ==
  In1 : Inport
  Memory1 : Memory
  Memory3 : Memory
  Multiply : Gain  Gain=0.0005
  NOT1 : Logic  Operator=NOT  IconShape=distinctive  AllPortsSameDT=off  OutDataTypeStr=boolean
  OR : Logic  Operator=OR  IconShape=distinctive  AllPortsSameDT=off  OutDataTypeStr=boolean
  One : Constant  OutDataTypeStr=Inherit: Inherit via back propagation
  Product1 : Product
  Scope4 : Scope  NumInputPorts=4
  Switch1 : Switch  Threshold=1  SaturateOnIntegerOverflow=off  InputSameDT=off
  Triggered Subsystem1 : Subsystem  TreatAsAtomicUnit=on
  Zero : Constant  Value=0  OutDataTypeStr=Inherit: Inherit via back propagation
  clock : Outport
  wires:
  Product1/1 -> Multiply/1, Memory1/1, Scope4/2
  One/1 -> Switch1/1
  Multiply/1 -> Switch1/2
  Triggered Subsystem1/1(Out1) -> Product1/1
  In1/1 -> Triggered Subsystem1/Trigger, Scope4/1
  Zero/1 -> Switch1/3
  NOT1/1 -> Product1/2
  Memory3/1 -> OR/2, NOT1/1
  Memory1/1 -> Triggered Subsystem1/1(In1)
  OR/1 -> Scope4/4, clock/1
  Switch1/1 -> Scope4/3, Memory3/1, OR/1

== system pattern3x3_training_2023clock/Post_Neuron3/Subsystem3/spike_generator2 ==
  del_th : Inport
  AND : Logic  IconShape=distinctive  AllPortsSameDT=off  OutDataTypeStr=boolean
  Delay1 : Delay  DelayLength=1  SampleTime=0.00001
  NOT : Logic  Operator=NOT  IconShape=distinctive  AllPortsSameDT=off  OutDataTypeStr=boolean
  Product : Product
  del_th_spike : Outport
  wires:
  NOT/1 -> Delay1/1
  AND/1 -> Product/1
  Delay1/1 -> AND/2
  Product/1 -> del_th_spike/1
  del_th/1 -> AND/1, Product/2, NOT/1

== system pattern3x3_training_2023clock/Post_Neuron4/Clock1/Triggered Subsystem1 ==
  In1 : Inport
  Trigger : TriggerPort  VariantControl=Variant
  Constant : Constant
  Sum : Sum  Inputs=|++
  Out1 : Outport  VectorParamsAs1DForOutWhenUnconnected=off
  wires:
  Constant/1 -> Sum/2
  In1/1 -> Sum/1
  Sum/1 -> Out1/1

== system pattern3x3_training_2023clock/Post_Neuron4/Clock2/Triggered Subsystem1 ==
  In1 : Inport
  Trigger : TriggerPort  VariantControl=Variant
  Constant : Constant
  Sum : Sum  Inputs=|++
  Out1 : Outport  VectorParamsAs1DForOutWhenUnconnected=off
  wires:
  Constant/1 -> Sum/2
  In1/1 -> Sum/1
  Sum/1 -> Out1/1

== system pattern3x3_training_2023clock/Post_Neuron4/Subsystem3/clock_0.02 ==
  In1 : Inport
  Memory1 : Memory
  Memory3 : Memory
  Multiply : Gain  Gain=0.0005
  NOT1 : Logic  Operator=NOT  IconShape=distinctive  AllPortsSameDT=off  OutDataTypeStr=boolean
  OR : Logic  Operator=OR  IconShape=distinctive  AllPortsSameDT=off  OutDataTypeStr=boolean
  One : Constant  OutDataTypeStr=Inherit: Inherit via back propagation
  Product1 : Product
  Scope4 : Scope  NumInputPorts=4
  Switch1 : Switch  Threshold=1  SaturateOnIntegerOverflow=off  InputSameDT=off
  Triggered Subsystem1 : Subsystem  TreatAsAtomicUnit=on
  Zero : Constant  Value=0  OutDataTypeStr=Inherit: Inherit via back propagation
  clock : Outport
  wires:
  Product1/1 -> Multiply/1, Memory1/1, Scope4/2
  One/1 -> Switch1/1
  Multiply/1 -> Switch1/2
  Triggered Subsystem1/1(Out1) -> Product1/1
  In1/1 -> Triggered Subsystem1/Trigger, Scope4/1
  Zero/1 -> Switch1/3
  NOT1/1 -> Product1/2
  Memory3/1 -> OR/2, NOT1/1
  Memory1/1 -> Triggered Subsystem1/1(In1)
  OR/1 -> Scope4/4, clock/1
  Switch1/1 -> Scope4/3, Memory3/1, OR/1

== system pattern3x3_training_2023clock/Post_Neuron4/Subsystem3/spike_generator2 ==
  del_th : Inport
  AND : Logic  IconShape=distinctive  AllPortsSameDT=off  OutDataTypeStr=boolean
  Delay1 : Delay  DelayLength=1  SampleTime=0.00001
  NOT : Logic  Operator=NOT  IconShape=distinctive  AllPortsSameDT=off  OutDataTypeStr=boolean
  Product : Product
  del_th_spike : Outport
  wires:
  NOT/1 -> Delay1/1
  AND/1 -> Product/1
  Delay1/1 -> AND/2
  Product/1 -> del_th_spike/1
  del_th/1 -> AND/1, Product/2, NOT/1

== system pattern3x3_training_2023clock/Synapse1/Clock1/Triggered Subsystem1 ==
  In1 : Inport
  Trigger : TriggerPort  VariantControl=Variant
  Constant : Constant
  Sum : Sum  Inputs=|++
  Out1 : Outport  VectorParamsAs1DForOutWhenUnconnected=off
  wires:
  Constant/1 -> Sum/2
  In1/1 -> Sum/1
  Sum/1 -> Out1/1

== system pattern3x3_training_2023clock/Synapse1/Clock2/Triggered Subsystem1 ==
  In1 : Inport
  Trigger : TriggerPort  VariantControl=Variant
  Constant : Constant
  Sum : Sum  Inputs=|++
  Out1 : Outport  VectorParamsAs1DForOutWhenUnconnected=off
  wires:
  Constant/1 -> Sum/2
  In1/1 -> Sum/1
  Sum/1 -> Out1/1

== system pattern3x3_training_2023clock/Synapse1/Clock3/Triggered Subsystem1 ==
  In1 : Inport
  Trigger : TriggerPort  VariantControl=Variant
  Constant : Constant
  Sum : Sum  Inputs=|++
  Out1 : Outport  VectorParamsAs1DForOutWhenUnconnected=off
  wires:
  Constant/1 -> Sum/2
  In1/1 -> Sum/1
  Sum/1 -> Out1/1

== system pattern3x3_training_2023clock/Synapse10/Clock1/Triggered Subsystem1 ==
  In1 : Inport
  Trigger : TriggerPort  VariantControl=Variant
  Constant : Constant
  Sum : Sum  Inputs=|++
  Out1 : Outport  VectorParamsAs1DForOutWhenUnconnected=off
  wires:
  Constant/1 -> Sum/2
  In1/1 -> Sum/1
  Sum/1 -> Out1/1

== system pattern3x3_training_2023clock/Synapse10/Clock2/Triggered Subsystem1 ==
  In1 : Inport
  Trigger : TriggerPort  VariantControl=Variant
  Constant : Constant
  Sum : Sum  Inputs=|++
  Out1 : Outport  VectorParamsAs1DForOutWhenUnconnected=off
  wires:
  Constant/1 -> Sum/2
  In1/1 -> Sum/1
  Sum/1 -> Out1/1

== system pattern3x3_training_2023clock/Synapse10/Clock3/Triggered Subsystem1 ==
  In1 : Inport
  Trigger : TriggerPort  VariantControl=Variant
  Constant : Constant
  Sum : Sum  Inputs=|++
  Out1 : Outport  VectorParamsAs1DForOutWhenUnconnected=off
  wires:
  Constant/1 -> Sum/2
  In1/1 -> Sum/1
  Sum/1 -> Out1/1

== system pattern3x3_training_2023clock/Synapse11/Clock1/Triggered Subsystem1 ==
  In1 : Inport
  Trigger : TriggerPort  VariantControl=Variant
  Constant : Constant
  Sum : Sum  Inputs=|++
  Out1 : Outport  VectorParamsAs1DForOutWhenUnconnected=off
  wires:
  Constant/1 -> Sum/2
  In1/1 -> Sum/1
  Sum/1 -> Out1/1

== system pattern3x3_training_2023clock/Synapse11/Clock2/Triggered Subsystem1 ==
  In1 : Inport
  Trigger : TriggerPort  VariantControl=Variant
  Constant : Constant
  Sum : Sum  Inputs=|++
  Out1 : Outport  VectorParamsAs1DForOutWhenUnconnected=off
  wires:
  Constant/1 -> Sum/2
  In1/1 -> Sum/1
  Sum/1 -> Out1/1

== system pattern3x3_training_2023clock/Synapse11/Clock3/Triggered Subsystem1 ==
  In1 : Inport
  Trigger : TriggerPort  VariantControl=Variant
  Constant : Constant
  Sum : Sum  Inputs=|++
  Out1 : Outport  VectorParamsAs1DForOutWhenUnconnected=off
  wires:
  Constant/1 -> Sum/2
  In1/1 -> Sum/1
  Sum/1 -> Out1/1

== system pattern3x3_training_2023clock/Synapse12/Clock1/Triggered Subsystem1 ==
  In1 : Inport
  Trigger : TriggerPort  VariantControl=Variant
  Constant : Constant
  Sum : Sum  Inputs=|++
  Out1 : Outport  VectorParamsAs1DForOutWhenUnconnected=off
  wires:
  Constant/1 -> Sum/2
  In1/1 -> Sum/1
  Sum/1 -> Out1/1

== system pattern3x3_training_2023clock/Synapse12/Clock2/Triggered Subsystem1 ==
  In1 : Inport
  Trigger : TriggerPort  VariantControl=Variant
  Constant : Constant
  Sum : Sum  Inputs=|++
  Out1 : Outport  VectorParamsAs1DForOutWhenUnconnected=off
  wires:
  Constant/1 -> Sum/2
  In1/1 -> Sum/1
  Sum/1 -> Out1/1
